simulink model "Test_Arithmetic_Operation_Bit_Adder_Carry_Out"  (Simulink 8.7)
settings: Solver=ode45  StartTime=0.0  StopTime=len  RelTol=1e-3
libraries: Arithmetic_Operations_Lib x1
settings Model: Creator=uzivatel  LastModifiedBy=Jozko Mrkvicka
settings DebuggingCC: SolverPrmCheckMsg=warning  StateNameClashWarn=warning

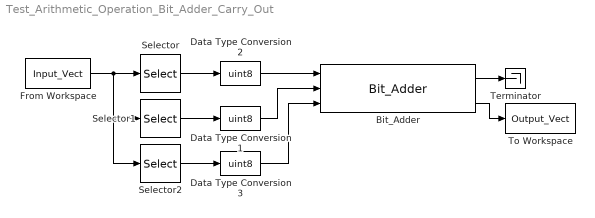
== system Test_Arithmetic_Operation_Bit_Adder_Carry_Out ==
  Bit_Adder : Arithmetic_Operations_Lib/Arithmetic_Operations_Lib/Bit_Adder
  Data Type Conversion1 : DataTypeConversion  OutDataTypeStr=uint8
  Data Type Conversion2 : DataTypeConversion  OutDataTypeStr=uint8
  Data Type Conversion3 : DataTypeConversion  OutDataTypeStr=uint8
  From Workspace : FromWorkspace  VariableName=Input_Vect  SampleTime=1  Interpolate=off  OutputAfterFinalValue=Holding final value
  Selector : Selector  IndexMode=Zero-based  InputPortWidth=3  SampleTime=1  IndexOptions=Index vector (dialog)  Indices=0  OutputSizes=1
  Selector1 : Selector  IndexMode=Zero-based  InputPortWidth=3  SampleTime=1  IndexOptions=Index vector (dialog)  Indices=1  OutputSizes=1
  Selector2 : Selector  IndexMode=Zero-based  InputPortWidth=3  SampleTime=1  IndexOptions=Index vector (dialog)  Indices=2  OutputSizes=1
  Terminator : Terminator
  To Workspace : ToWorkspace  VariableName=Output_Vect  SampleTime=1
  wires:
  From Workspace/1 -> Selector2/1, Selector1/1, Selector/1
  Selector1/1 -> Data Type Conversion1/1
  Selector/1 -> Data Type Conversion2/1
  Data Type Conversion2/1 -> Bit_Adder/1
  Bit_Adder/1 -> Terminator/1
  Bit_Adder/2 -> To Workspace/1
  Selector2/1 -> Data Type Conversion3/1
  Data Type Conversion1/1 -> Bit_Adder/2
  Data Type Conversion3/1 -> Bit_Adder/3
